simulink model "sigma2nd_d"  (Simulink 7.4)
settings: Solver=ode23t  StartTime=0.0  StopTime=70e-3  MaxStep=1e-6  RelTol=1e-3
PreLoadFcn:
  | Fs=512e3;
  | N=4;   % Number of CIC stages
  | R=16;  % Decimation factor
  | M=1;   % Delay order
  | b=ones(R*M,1)/(R*M);                % Compensate for gain of CIC for analysis purposes.
  | CICnum = conv(b,conv(b,conv(b,b)));  % overall cic numerator
  | load d4_coeff;
StartFcn:
  | tic
StopFcn:
  | trun=toc
undefined symbols (not defined in the file or in its folder): One, sided
libraries: powerlib x72, dspmlti4 x2, simulink x2, dspsnks4 x1
settings Model: Creator=dbenson  LastModifiedBy=Dick
settings DataIOCC: SaveOutput=off  SaveTime=off  SignalLoggingName=sigsOut
settings OptimizationCC: InlineInvariantSignals=on  InitFltsAndDblsToZero=on
settings DebuggingCC: SaveWithParameterizedLinksMsg=none  SignalResolutionControl=TryResolveAllWithWarning  SolverPrmCheckMsg=none  MultiTaskDSMMsg=warning  MultiTaskCondExecSysMsg=none  UnconnectedLineMsg=none  StrictBusMsg=None
settings HardwareCC: TargetUnknown=on
settings RTWCC: IncludeERTFirstTime=on
settings GRTTargetCC: TargetFcnLib=ansi_tfl_tmw.mat

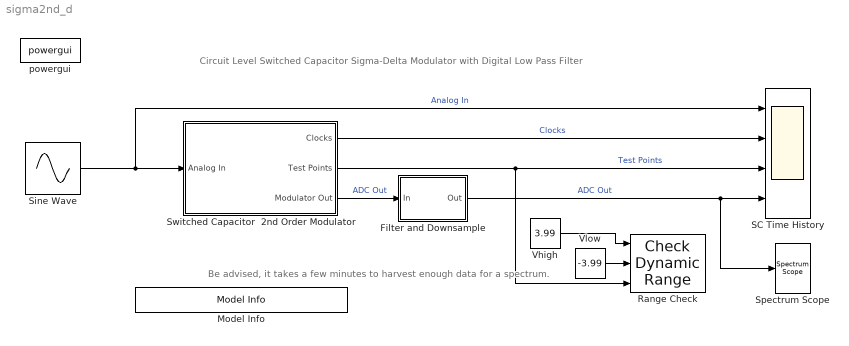
== system sigma2nd_d ==
  note: Circuit Level Switched Capacitor Sigma-Delta Modulator
      | with
      | Digital Low Pass Filter
  note: Be advised, it takes a few minutes
      |  to harvest enough data for a spectrum.
  Filter and Downsample : Subsystem
  Model Info : simulink/Model-Wide Utilities/Model Info  SystemSampleTime=-1  InitialBlockCM=None  BlockCM=None  Frame=on  DisplayStringWithTags=Copywrite 2005-2010 The MathWorks, Inc.  HorizontalTextAlignment=Center  LeftAlignmentValue=0.5  SourceBlockDiagram=sigma2nd_d  TagMaxNumber=20
  Range Check : simulink/Model Verification/Check  Dynamic Range  Description=min < sig < max  SystemSampleTime=-1  enabled=on  stopWhenAssertionFail=off  export=off  icon=graphic
  SC Time History : Scope  NumInputPorts=4
      settings: TimeRange=0.0025  YMin=-0.5~-0.2~-4~-0.5  YMax=0.5~1.2~4~0.5  DataFormat=Structure  Decimation=40
  Sine Wave : Sin  Amplitude=0.45  Bias=0  Frequency=500*2*pi  Phase=0  Samples=10  SampleTime=0  Offset=0
  Spectrum Scope : dspsnks4/Spectrum Scope  DialogController=dspdialog.SpectrumScope  DialogControllerArgs=DataTag2  SystemSampleTime=-1  ScopeProperties=on  Domain=Frequency  HorizSpan=1  UseBuffer=on  BufferSize=512  Overlap=0  inpFftLenInherit=off  FFTlength=128  numAvg=1  DisplayProperties=off  AxisGrid=on  Memory=off  FrameNumber=on  AxisLegend=off  AxisZoom=off  OpenScopeAtSimStart=on  OpenScopeImmediately=off  FigPos=[444 39 414 275]  AxisProperties=off  XUnits=Hertz  XRange=One-sided ([0...Fs/2])  XDisplay=0  InheritXIncr=on  XIncr=64/Fs  XLabel=Samples  XLimit=Auto  YUnits=dBW  XMax=1  XMin=0  YLabel=dBW  LineProperties=off  wintypeSpecScope=Hann  RsSpecScope=50  betaSpecScope=5  winsampSpecScope=Periodic  XAxisParamsVer=6.9
      settings: YMin=-100  YMax=0
  Switched Capacitor  2nd Order Modulator : Subsystem
  Vhigh : Constant  Value=3.99  OutDataType=sfix(16)  OutScaling=2^0
  Vlow : Constant  Value=-3.99  OutDataType=sfix(16)  OutScaling=2^0
  powergui : powerlib/powergui  SystemSampleTime=-1  SimulationMode=Continuous  SampleTime=50e-6  frequency=60  SPID=off  DisableSnubberDevices=off  DisableRonSwitches=off  DisableVfSwitches=off  SwTol=0  Interpol=off  frequencyindice=0  echomessages=off  HookPort=off  DisplayEquations=off  FunctionMessages=off  EnableUseOfTLC=off  x0status=blocks  RestoreLinks=warning  Frange=[0:2:500]  Ylog=off  Xlog=on  ShowGrid=off  save=off  variable=ZData  ZoomFFT=on  StartTime=0.0  cycles=1  DisplayStyle=1  fundamental=60  FreqAxis=off  MaxFrequency=1000  frequencyindicesteady=1  RmsSteady=1  display=off  Ts=0  methode=off
  wires:
  Sine Wave/1 -> Switched Capacitor  2nd Order Modulator/1(Analog In), SC Time History/1  "Analog In"
  Switched Capacitor  2nd Order Modulator/3(Modulator Out) -> Filter and Downsample/1(In)  "ADC Out"
  Switched Capacitor  2nd Order Modulator/2(Test Points) -> Range Check/3, SC Time History/3  "Test Points"
  Vhigh/1 -> Range Check/1
  Vlow/1 -> Range Check/2
  Switched Capacitor  2nd Order Modulator/1(Clocks) -> SC Time History/2  "Clocks"
  Filter and Downsample/1(Out) -> SC Time History/4, Spectrum Scope/1  "ADC Out"

== system sigma2nd_d/Filter and Downsample ==
  In : Inport  OutDataType=sfix(16)  OutScaling=2^0
  D=16 Cascaded Integrator Comb Filter : dspmlti4/FIR Decimation  DialogController=dspdialog.FIRDecimation  DialogControllerArgs=DataTag0  h=CICnum  D=16  filtStruct=Direct form  framing=Maintain input frame size  outputBufInitCond=0  roundingMode=Floor  overflowMode=off  FilterSource=Specify via dialog  FilterObject=Hm_firdecim
  "D=4 with inverse sinc correction " : dspmlti4/FIR Decimation  DialogController=dspdialog.FIRDecimation  DialogControllerArgs=DataTag1  h=d4_coeff  D=4  filtStruct=Direct form  framing=Maintain input frame size  outputBufInitCond=0  roundingMode=Floor  overflowMode=off  FilterSource=Specify via dialog  FilterObject=Hm_firdecim
  Out : Outport  OutDataType=sfix(16)  OutScaling=2^0
  wires:
  "D=4 with inverse sinc correction "/1 -> Out/1
  In/1 -> D=16 Cascaded Integrator Comb Filter/1
  D=16 Cascaded Integrator Comb Filter/1 -> "D=4 with inverse sinc correction "/1

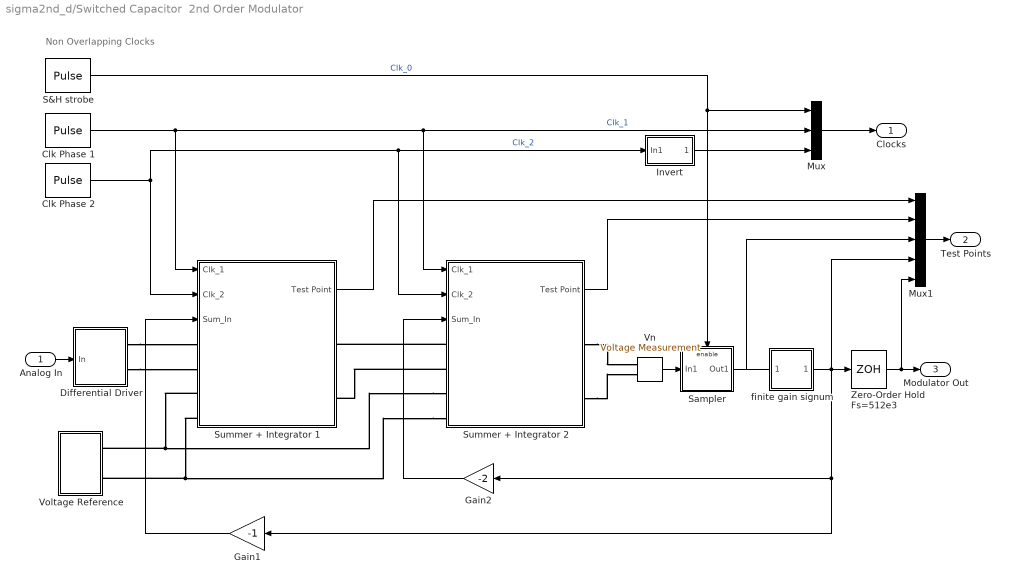
== system sigma2nd_d/Switched Capacitor  2nd Order Modulator ==
  note: Non Overlapping Clocks
  Analog In : Inport  OutDataType=sfix(16)  OutScaling=2^0
  Clk Phase 1 : DiscretePulseGenerator  PulseType=Time based  Amplitude=1  Period=1/Fs  PulseWidth=49.9  PhaseDelay=0.001/Fs  SampleTime=1
  Clk Phase 2 : DiscretePulseGenerator  PulseType=Time based  Amplitude=1  Period=1/Fs  PulseWidth=50.1  PhaseDelay=0  SampleTime=1
  Differential Driver : Subsystem
  Gain1 : Gain  Gain=-1  ParameterDataType=sfix(16)  ParameterScaling=2^0  OutDataType=sfix(16)  OutScaling=2^0  SaturateOnIntegerOverflow=on  OutDataTypeStr=Inherit: Same as input  ParamDataTypeStr=Inherit: Same as input
  Gain2 : Gain  Gain=-2  ParameterDataType=sfix(16)  ParameterScaling=2^0  OutDataType=sfix(16)  OutScaling=2^0  SaturateOnIntegerOverflow=on  OutDataTypeStr=Inherit: Same as input  ParamDataTypeStr=Inherit: Same as input
  Invert : Subsystem
  Mux : Mux  Inputs=3
  Mux1 : Mux  Inputs=5
  S&H strobe : DiscretePulseGenerator  PulseType=Time based  Amplitude=1  Period=1/Fs  PulseWidth=0.01  PhaseDelay=0.5005/Fs  SampleTime=1
  Sampler : Subsystem
  Summer + Integrator 1 : Subsystem
  Summer + Integrator 2 : Subsystem
  "Vn " : powerlib/Measurements/Voltage Measurement  Tag=PoWeRsYsTeMmEaSuReMeNt  DialogController=POWERSYS.PowerSysDialog  SystemSampleTime=-1  PhasorSimulation=off  OutputType=Magnitude  PSBequivalent=0
  Voltage Reference : Subsystem
  "Zero-Order Hold  Fs=512e3 " : ZeroOrderHold  SampleTime=1/Fs
  "finite gain signum " : Subsystem  mask{alpha=1e6}
      mask init:
      | x=-3:0.05:3;  y= tanh(alpha*x);
      mask Display: plot(x,y)
  Clocks : Outport  OutDataType=sfix(16)  OutScaling=2^0
  Test Points : Outport  Port=2  OutDataType=sfix(16)  OutScaling=2^0
  Modulator Out : Outport  Port=3  OutDataType=sfix(16)  OutScaling=2^0
  wires:
  Clk Phase 1/1 -> Summer + Integrator 1/1(Clk_1), Mux/2, Summer + Integrator 2/1(Clk_1)  "Clk_1"
  Clk Phase 2/1 -> Summer + Integrator 1/2(Clk_2), Summer + Integrator 2/2(Clk_2), Invert/1(In1)  "Clk_2"
  "Vn "/1 -> Sampler/1(In1)
  Gain1/1 -> Summer + Integrator 1/3(Sum_In)
  Analog In/1 -> Differential Driver/1(In)
  Mux/1 -> Clocks/1
  S&H strobe/1 -> Mux/1, Sampler/Enable  "Clk_0"
  Gain2/1 -> Summer + Integrator 2/3(Sum_In)
  Mux1/1 -> Test Points/1
  Sampler/1(Out1) -> "finite gain signum "/1(In1), Mux1/3
  "Zero-Order Hold  Fs=512e3 "/1 -> Modulator Out/1, Mux1/5
  Invert/1(Out1) -> Mux/3
  Summer + Integrator 1/1(Test Point) -> Mux1/1
  Summer + Integrator 2/1(Test Point) -> Mux1/2
  "finite gain signum "/1(Out1) -> Mux1/4, "Zero-Order Hold  Fs=512e3 "/1, Gain2/1, Gain1/1
  connections:
  Summer + Integrator 2/LConn3 -- Voltage Reference/RConn1 -- Summer + Integrator 1/LConn3
  Summer + Integrator 2/LConn4 -- Summer + Integrator 1/LConn4 -- Voltage Reference/RConn2
  Differential Driver/RConn1 -- Summer + Integrator 1/LConn1
  Differential Driver/RConn2 -- Summer + Integrator 1/LConn2
  Summer + Integrator 2/RConn2 -- "Vn "/LConn2
  Summer + Integrator 2/RConn1 -- "Vn "/LConn1
  Summer + Integrator 2/LConn1 -- Summer + Integrator 1/RConn1
  Summer + Integrator 2/LConn2 -- Summer + Integrator 1/RConn2

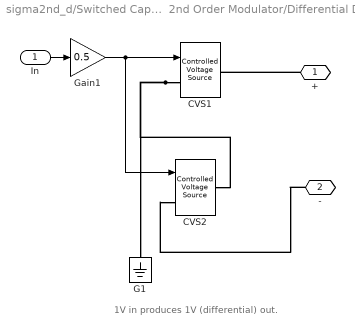
== system sigma2nd_d/Switched Capacitor  2nd Order Modulator/Differential Driver ==
  note: 1V in produces 1V (differential) out.
  In : Inport  OutDataType=sfix(16)  OutScaling=2^0
  CVS1 : powerlib/Electrical Sources/Controlled Voltage Source  Description=source block  DialogController=POWERSYS.PowerSysDialog  SystemSampleTime=-1  Initialize=off  Source_Type=AC  Amplitude=0  Phase=0  Frequency=0  Measurements=None
      settings: AttributesFormatString=\n
  CVS2 : powerlib/Electrical Sources/Controlled Voltage Source  Description=source block  DialogController=POWERSYS.PowerSysDialog  SystemSampleTime=-1  Initialize=off  Source_Type=AC  Amplitude=0  Phase=0  Frequency=0  Measurements=None
      settings: AttributesFormatString=\n
  G1 : powerlib/Elements/Ground  DialogController=POWERSYS.PowerSysDialog  PhysicalDomain=powersysdomain  SubClassName=unknown  LeftPortType=p1  RightPortType=p1  LConnTagsString=a
  Gain1 : Gain  Gain=0.5  ParameterDataType=sfix(16)  ParameterScaling=2^0  OutDataType=sfix(16)  OutScaling=2^0  SaturateOnIntegerOverflow=on  OutDataTypeStr=Inherit: Same as input  ParamDataTypeStr=Inherit: Same as input
  + : PMIOPort  Port=1  Side=Right
  - : PMIOPort  Port=2  Side=Right
  wires:
  In/1 -> Gain1/1
  Gain1/1 -> CVS1/1, CVS2/1
  connections:
  CVS1/LConn1 -- CVS2/RConn1 -- G1/LConn1
  +/RConn1 -- CVS1/RConn1
  -/RConn1 -- CVS2/LConn1

== system sigma2nd_d/Switched Capacitor  2nd Order Modulator/Invert ==
  In1 : Inport  OutDataType=sfix(16)  OutScaling=2^0
  Data Type Conversion : DataTypeConversion  OutDataTypeMode=boolean  OutDataType=sfix(16)  OutScaling=2^0  OutDataTypeStr=boolean  SaturateOnIntegerOverflow=on  RndMeth=Zero
  Data Type Conversion1 : DataTypeConversion  OutDataTypeMode=double  OutDataType=sfix(16)  OutScaling=2^0  OutDataTypeStr=double  SaturateOnIntegerOverflow=on  RndMeth=Zero
  Logical Operator : Logic  Operator=NOT  AllPortsSameDT=off
  Out1 : Outport  OutDataType=sfix(16)  OutScaling=2^0
  wires:
  Data Type Conversion/1 -> Logical Operator/1
  Logical Operator/1 -> Data Type Conversion1/1
  In1/1 -> Data Type Conversion/1
  Data Type Conversion1/1 -> Out1/1

== system sigma2nd_d/Switched Capacitor  2nd Order Modulator/Sampler ==
  In1 : Inport  OutDataType=sfix(16)  OutScaling=2^0
  Enable : EnablePort
  Out1 : Outport  OutDataType=sfix(16)  OutScaling=2^0  InitialOutput=[0]
  wires:
  In1/1 -> Out1/1

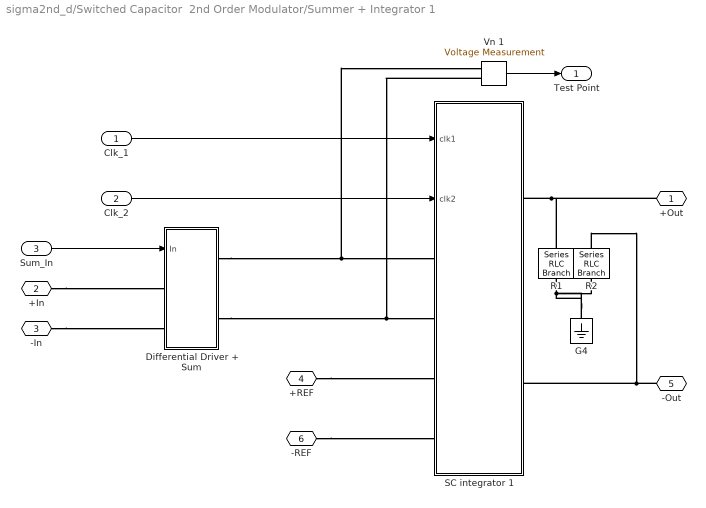
== system sigma2nd_d/Switched Capacitor  2nd Order Modulator/Summer + Integrator 1 ==
  Clk_1 : Inport  OutDataType=sfix(16)  OutScaling=2^0
  Clk_2 : Inport  Port=2  OutDataType=sfix(16)  OutScaling=2^0
  Sum_In : Inport  Port=3  OutDataType=sfix(16)  OutScaling=2^0
  Differential Driver + Sum : Subsystem
  G4 : powerlib/Elements/Ground  DialogController=POWERSYS.PowerSysDialog  PhysicalDomain=powersysdomain  SubClassName=unknown  LeftPortType=p1  RightPortType=p1  LConnTagsString=a
  R1 : powerlib/Elements/Series RLC Branch  DialogController=POWERSYS.PowerSysDialog  PhysicalDomain=powersysdomain  SubClassName=unknown  LeftPortType=p1  RightPortType=p1  LConnTagsString=__new0  RConnTagsString=__new0  BranchType=R  Resistance=1e9  Inductance=1.0  SetiL0=off  InitialCurrent=0  Capacitance=1.0  Setx0=off  InitialVoltage=0  Measurements=None
  R2 : powerlib/Elements/Series RLC Branch  DialogController=POWERSYS.PowerSysDialog  PhysicalDomain=powersysdomain  SubClassName=unknown  LeftPortType=p1  RightPortType=p1  LConnTagsString=__new0  RConnTagsString=__new0  BranchType=R  Resistance=1e9  Inductance=1.0  SetiL0=off  InitialCurrent=0  Capacitance=1.0  Setx0=off  InitialVoltage=0  Measurements=None
  SC integrator 1 : Subsystem  mask{Ci=4e-12, Cs=2e-12, Ron=10, Fb1=1e9, Fb2=1e8, Avol=2000, Vs=4, Slew=inf}
      mask prompts: Ci "integrating Cap"; Cs "Sampling Cap"; Ron "Switch on resistor"
  Vn 1 : powerlib/Measurements/Voltage Measurement  Tag=PoWeRsYsTeMmEaSuReMeNt  DialogController=POWERSYS.PowerSysDialog  SystemSampleTime=-1  PhasorSimulation=off  OutputType=Magnitude  PSBequivalent=0
  +Out : PMIOPort  Port=1  Side=Right
  +In : PMIOPort  Port=2  Side=Left
  -In : PMIOPort  Port=3  Side=Left
  +REF : PMIOPort  Port=4  Side=Left
  -Out : PMIOPort  Port=5  Side=Right
  -REF : PMIOPort  Port=6  Side=Left
  Test Point : Outport  OutDataType=sfix(16)  OutScaling=2^0
  wires:
  Clk_1/1 -> SC integrator 1/1(clk1)
  Clk_2/1 -> SC integrator 1/2(clk2)
  Sum_In/1 -> Differential Driver + Sum/1(In)
  Vn 1/1 -> Test Point/1
  connections:
  Differential Driver + Sum/RConn1 -- SC integrator 1/LConn1 -- Vn 1/LConn1
  Vn 1/LConn2 -- SC integrator 1/LConn2 -- Differential Driver + Sum/RConn2
  +Out/RConn1 -- SC integrator 1/RConn1 -- R1/RConn1
  +REF/RConn1 -- SC integrator 1/LConn3
  -Out/RConn1 -- SC integrator 1/RConn2 -- R2/RConn1
  -REF/RConn1 -- SC integrator 1/LConn4
  +In/RConn1 -- Differential Driver + Sum/LConn1
  -In/RConn1 -- Differential Driver + Sum/LConn2
  R1/LConn1 -- G4/LConn1 -- R2/LConn1

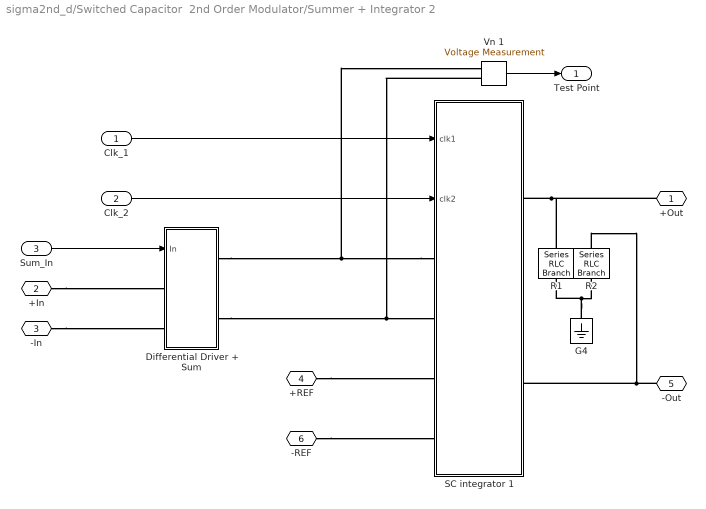
== system sigma2nd_d/Switched Capacitor  2nd Order Modulator/Summer + Integrator 2 ==
  Clk_1 : Inport  OutDataType=sfix(16)  OutScaling=2^0
  Clk_2 : Inport  Port=2  OutDataType=sfix(16)  OutScaling=2^0
  Sum_In : Inport  Port=3  OutDataType=sfix(16)  OutScaling=2^0
  Differential Driver + Sum : Subsystem
  G4 : powerlib/Elements/Ground  DialogController=POWERSYS.PowerSysDialog  PhysicalDomain=powersysdomain  SubClassName=unknown  LeftPortType=p1  RightPortType=p1  LConnTagsString=a
  R1 : powerlib/Elements/Series RLC Branch  DialogController=POWERSYS.PowerSysDialog  PhysicalDomain=powersysdomain  SubClassName=unknown  LeftPortType=p1  RightPortType=p1  LConnTagsString=__new0  RConnTagsString=__new0  BranchType=R  Resistance=1e9  Inductance=1.0  SetiL0=off  InitialCurrent=0  Capacitance=1.0  Setx0=off  InitialVoltage=0  Measurements=None
  R2 : powerlib/Elements/Series RLC Branch  DialogController=POWERSYS.PowerSysDialog  PhysicalDomain=powersysdomain  SubClassName=unknown  LeftPortType=p1  RightPortType=p1  LConnTagsString=__new0  RConnTagsString=__new0  BranchType=R  Resistance=1e9  Inductance=1.0  SetiL0=off  InitialCurrent=0  Capacitance=1.0  Setx0=off  InitialVoltage=0  Measurements=None
  SC integrator 1 : Subsystem  mask{Ci=4e-12, Cs=2e-12, Ron=10, Fb1=1e9, Fb2=1e8, Avol=2000, Vs=4, Slew=inf}
      mask prompts: Ci "integrating Cap"; Cs "Sampling Cap"; Ron "Switch on resistor"
  Vn 1 : powerlib/Measurements/Voltage Measurement  Tag=PoWeRsYsTeMmEaSuReMeNt  DialogController=POWERSYS.PowerSysDialog  SystemSampleTime=-1  PhasorSimulation=off  OutputType=Magnitude  PSBequivalent=0
  +Out : PMIOPort  Port=1  Side=Right
  +In : PMIOPort  Port=2  Side=Left
  -In : PMIOPort  Port=3  Side=Left
  +REF : PMIOPort  Port=4  Side=Left
  -Out : PMIOPort  Port=5  Side=Right
  -REF : PMIOPort  Port=6  Side=Left
  Test Point : Outport  OutDataType=sfix(16)  OutScaling=2^0
  wires:
  Vn 1/1 -> Test Point/1
  Sum_In/1 -> Differential Driver + Sum/1(In)
  Clk_2/1 -> SC integrator 1/2(clk2)
  Clk_1/1 -> SC integrator 1/1(clk1)
  connections:
  G4/LConn1 -- R1/LConn1 -- R2/LConn1
  -In/RConn1 -- Differential Driver + Sum/LConn2
  +In/RConn1 -- Differential Driver + Sum/LConn1
  -REF/RConn1 -- SC integrator 1/LConn4
  R2/RConn1 -- SC integrator 1/RConn2 -- -Out/RConn1
  +REF/RConn1 -- SC integrator 1/LConn3
  R1/RConn1 -- SC integrator 1/RConn1 -- +Out/RConn1
  Differential Driver + Sum/RConn2 -- SC integrator 1/LConn2 -- Vn 1/LConn2
  SC integrator 1/LConn1 -- Differential Driver + Sum/RConn1 -- Vn 1/LConn1

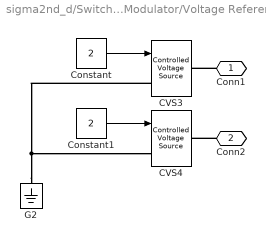
== system sigma2nd_d/Switched Capacitor  2nd Order Modulator/Voltage Reference ==
  CVS3 : powerlib/Electrical Sources/Controlled Voltage Source  Description=source block  DialogController=POWERSYS.PowerSysDialog  SystemSampleTime=-1  Initialize=off  Source_Type=AC  Amplitude=0  Phase=0  Frequency=0  Measurements=None
      settings: AttributesFormatString=\n
  CVS4 : powerlib/Electrical Sources/Controlled Voltage Source  Description=source block  DialogController=POWERSYS.PowerSysDialog  SystemSampleTime=-1  Initialize=off  Source_Type=AC  Amplitude=0  Phase=0  Frequency=0  Measurements=None
      settings: AttributesFormatString=\n
  Constant : Constant  Value=2  OutDataType=sfix(16)  OutScaling=2^0
  Constant1 : Constant  Value=2  OutDataType=sfix(16)  OutScaling=2^0
  G2 : powerlib/Elements/Ground  DialogController=POWERSYS.PowerSysDialog  PhysicalDomain=powersysdomain  SubClassName=unknown  LeftPortType=p1  RightPortType=p1  LConnTagsString=a
  Conn1 : PMIOPort  Port=1  Side=Right
  Conn2 : PMIOPort  Port=2  Side=Right
  wires:
  Constant/1 -> CVS3/1
  Constant1/1 -> CVS4/1
  connections:
  CVS3/LConn1 -- G2/LConn1 -- CVS4/LConn1
  Conn1/RConn1 -- CVS3/RConn1
  Conn2/RConn1 -- CVS4/RConn1

== system sigma2nd_d/Switched Capacitor  2nd Order Modulator/finite gain signum  ==
  In1 : Inport  OutDataType=sfix(16)  OutScaling=2^0
  Gain1 : Gain  Gain=alpha  ParameterDataType=sfix(16)  ParameterScaling=2^0  OutDataType=sfix(16)  OutScaling=2^0  SaturateOnIntegerOverflow=on  OutDataTypeStr=Inherit: Same as input  ParamDataTypeStr=Inherit: Same as input
  Hyperbolic Tangent : Trigonometry  Operator=tanh
  Memory : Memory
  Out1 : Outport  OutDataType=sfix(16)  OutScaling=2^0
  wires:
  In1/1 -> Gain1/1
  Gain1/1 -> Hyperbolic Tangent/1
  Hyperbolic Tangent/1 -> Memory/1
  Memory/1 -> Out1/1

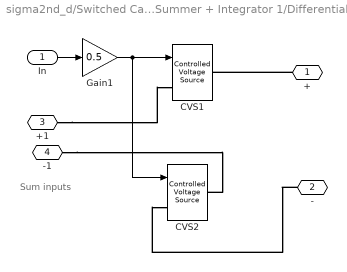
== system sigma2nd_d/Switched Capacitor  2nd Order Modulator/Summer + Integrator 1/Differential Driver + Sum ==
  note: Sum inputs
  In : Inport  OutDataType=sfix(16)  OutScaling=2^0
  CVS1 : powerlib/Electrical Sources/Controlled Voltage Source  Description=source block  DialogController=POWERSYS.PowerSysDialog  SystemSampleTime=-1  Initialize=off  Source_Type=AC  Amplitude=0  Phase=0  Frequency=0  Measurements=None
      settings: AttributesFormatString=\n
  CVS2 : powerlib/Electrical Sources/Controlled Voltage Source  Description=source block  DialogController=POWERSYS.PowerSysDialog  SystemSampleTime=-1  Initialize=off  Source_Type=AC  Amplitude=0  Phase=0  Frequency=0  Measurements=None
      settings: AttributesFormatString=\n
  Gain1 : Gain  Gain=0.5  ParameterDataType=sfix(16)  ParameterScaling=2^0  OutDataType=sfix(16)  OutScaling=2^0  SaturateOnIntegerOverflow=on  OutDataTypeStr=Inherit: Same as input  ParamDataTypeStr=Inherit: Same as input
  + : PMIOPort  Port=1  Side=Right
  - : PMIOPort  Port=2  Side=Right
  +1 : PMIOPort  Port=3  Side=Left
  -1 : PMIOPort  Port=4  Side=Left
  wires:
  In/1 -> Gain1/1
  Gain1/1 -> CVS1/1, CVS2/1
  connections:
  +/RConn1 -- CVS1/RConn1
  -/RConn1 -- CVS2/LConn1
  +1/RConn1 -- CVS1/LConn1
  -1/RConn1 -- CVS2/RConn1

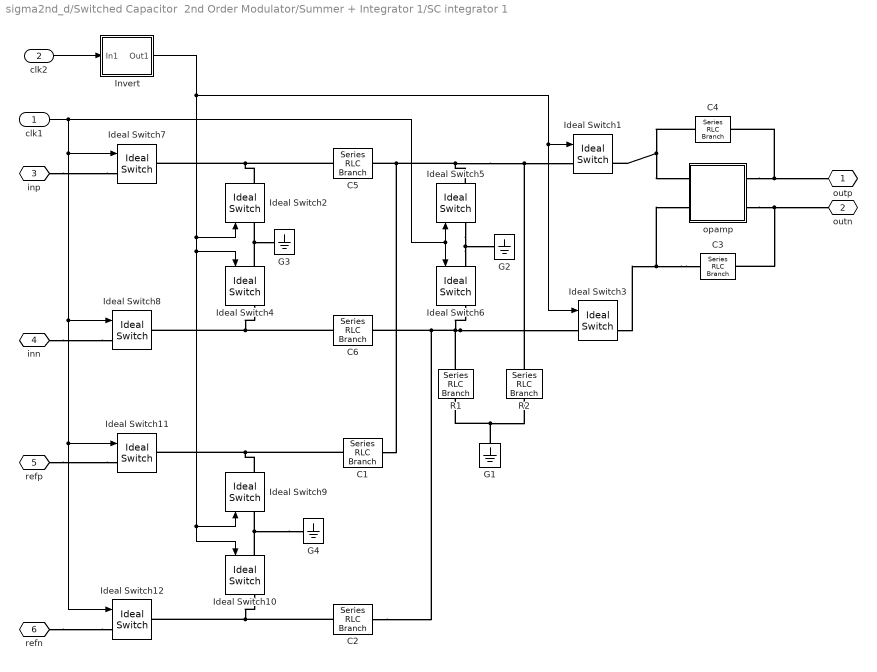
== system sigma2nd_d/Switched Capacitor  2nd Order Modulator/Summer + Integrator 1/SC integrator 1 ==
  clk1 : Inport  OutDataType=sfix(16)  OutScaling=2^0
  clk2 : Inport  Port=2  OutDataType=sfix(16)  OutScaling=2^0
  C{1..2,5..6} (4 alike) : powerlib/Elements/Series RLC Branch  DialogController=POWERSYS.PowerSysDialog  PhysicalDomain=powersysdomain  SubClassName=unknown  LeftPortType=p1  RightPortType=p1  LConnTagsString=__new0  RConnTagsString=__new0  BranchType=C  Resistance=1.0  Inductance=1.0  SetiL0=off  InitialCurrent=0  Capacitance=Cs  Setx0=off  InitialVoltage=0  Measurements=None
  C3 : powerlib/Elements/Series RLC Branch  DialogController=POWERSYS.PowerSysDialog  PhysicalDomain=powersysdomain  SubClassName=unknown  LeftPortType=p1  RightPortType=p1  LConnTagsString=__new0  RConnTagsString=__new0  BranchType=C  Resistance=1.0  Inductance=1.0  SetiL0=off  InitialCurrent=0  Capacitance=Ci  Setx0=off  InitialVoltage=0  Measurements=None
  "C4 " : powerlib/Elements/Series RLC Branch  DialogController=POWERSYS.PowerSysDialog  PhysicalDomain=powersysdomain  SubClassName=unknown  LeftPortType=p1  RightPortType=p1  LConnTagsString=__new0  RConnTagsString=__new0  BranchType=C  Resistance=1.0  Inductance=1.0  SetiL0=off  InitialCurrent=0  Capacitance=Ci  Setx0=off  InitialVoltage=0  Measurements=None
  G{1..4} (4 alike) : powerlib/Elements/Ground  DialogController=POWERSYS.PowerSysDialog  PhysicalDomain=powersysdomain  SubClassName=unknown  LeftPortType=p1  RightPortType=p1  LConnTagsString=a
  Ideal Switch{1..12} (12 alike) : powerlib/Power Electronics/Ideal Switch  DialogController=POWERSYS.PowerSysDialog  SystemSampleTime=-1  Ron=Ron  Lon=1e-9  IC=1  Rs=0  Cs=0  Measurements=off
      settings: AttributesFormatString=\n
  Invert : Subsystem
  R1 : powerlib/Elements/Series RLC Branch  DialogController=POWERSYS.PowerSysDialog  PhysicalDomain=powersysdomain  SubClassName=unknown  LeftPortType=p1  RightPortType=p1  LConnTagsString=__new0  RConnTagsString=__new0  BranchType=R  Resistance=1e9  Inductance=1.0  SetiL0=off  InitialCurrent=0  Capacitance=1.0  Setx0=off  InitialVoltage=0  Measurements=None
  R2 : powerlib/Elements/Series RLC Branch  DialogController=POWERSYS.PowerSysDialog  PhysicalDomain=powersysdomain  SubClassName=unknown  LeftPortType=p1  RightPortType=p1  LConnTagsString=__new0  RConnTagsString=__new0  BranchType=R  Resistance=1e9  Inductance=1.0  SetiL0=off  InitialCurrent=0  Capacitance=1.0  Setx0=off  InitialVoltage=0  Measurements=None
  opamp : Subsystem  mask{f2=Fb1, f1=Fb2, Av=Avol, v_min=-Vs, v_max=Vs, slew_rate=Slew}
      mask prompts: f2 "break freq 2 in Hz"; f1 "break freq 1 in Hz"; Av "Av (voltage gain)"; v_min "Min Output"; v_max "Max Output"; slew_rate "slew rate (v/s)"
      mask Display: plot([0 1 0 0] , [1 0 -1 1 ]); text(0.15,0.4,'+'); text(0.15,-0.4,'-');
  outp : PMIOPort  Port=1  Side=Right
  outn : PMIOPort  Port=2  Side=Right
  inp : PMIOPort  Port=3  Side=Left
  inn : PMIOPort  Port=4  Side=Left
  refp : PMIOPort  Port=5  Side=Left
  refn : PMIOPort  Port=6  Side=Left
  wires:
  Invert/1(Out1) -> Ideal Switch4/1, Ideal Switch9/1, Ideal Switch10/1, Ideal Switch2/1, Ideal Switch3/1, Ideal Switch1/1
  clk1/1 -> Ideal Switch12/1, Ideal Switch11/1, Ideal Switch8/1, Ideal Switch7/1, Ideal Switch5/1, Ideal Switch6/1
  clk2/1 -> Invert/1(In1)
  connections:
  refn/RConn1 -- Ideal Switch12/LConn1
  refp/RConn1 -- Ideal Switch11/LConn1
  inn/RConn1 -- Ideal Switch8/LConn1
  inp/RConn1 -- Ideal Switch7/LConn1
  G4/LConn1 -- Ideal Switch9/LConn1 -- Ideal Switch10/LConn1
  Ideal Switch2/LConn1 -- G3/LConn1 -- Ideal Switch4/LConn1
  Ideal Switch6/LConn1 -- G2/LConn1 -- Ideal Switch5/LConn1
  Ideal Switch11/RConn1 -- C1/LConn1 -- Ideal Switch9/RConn1
  Ideal Switch1/RConn1 -- opamp/LConn1 -- "C4 "/RConn1
  opamp/RConn1 -- outp/RConn1 -- "C4 "/LConn1
  C1/RConn1 -- C5/RConn1 -- Ideal Switch5/RConn1 -- Ideal Switch1/LConn1 -- R2/RConn1
  Ideal Switch2/RConn1 -- Ideal Switch7/RConn1 -- C5/LConn1
  C3/RConn1 -- opamp/LConn2 -- Ideal Switch3/RConn1
  opamp/RConn2 -- outn/RConn1 -- C3/LConn1
  Ideal Switch12/RConn1 -- C2/LConn1 -- Ideal Switch10/RConn1
  C2/RConn1 -- C6/RConn1 -- Ideal Switch6/RConn1 -- Ideal Switch3/LConn1 -- R1/RConn1
  Ideal Switch4/RConn1 -- Ideal Switch8/RConn1 -- C6/LConn1
  R2/LConn1 -- G1/LConn1 -- R1/LConn1

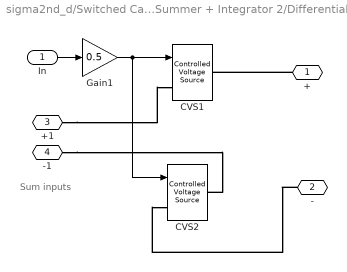
== system sigma2nd_d/Switched Capacitor  2nd Order Modulator/Summer + Integrator 2/Differential Driver + Sum ==
  note: Sum inputs
  In : Inport  OutDataType=sfix(16)  OutScaling=2^0
  CVS1 : powerlib/Electrical Sources/Controlled Voltage Source  Description=source block  DialogController=POWERSYS.PowerSysDialog  SystemSampleTime=-1  Initialize=off  Source_Type=AC  Amplitude=0  Phase=0  Frequency=0  Measurements=None
      settings: AttributesFormatString=\n
  CVS2 : powerlib/Electrical Sources/Controlled Voltage Source  Description=source block  DialogController=POWERSYS.PowerSysDialog  SystemSampleTime=-1  Initialize=off  Source_Type=AC  Amplitude=0  Phase=0  Frequency=0  Measurements=None
      settings: AttributesFormatString=\n
  Gain1 : Gain  Gain=0.5  ParameterDataType=sfix(16)  ParameterScaling=2^0  OutDataType=sfix(16)  OutScaling=2^0  SaturateOnIntegerOverflow=on  OutDataTypeStr=Inherit: Same as input  ParamDataTypeStr=Inherit: Same as input
  + : PMIOPort  Port=1  Side=Right
  - : PMIOPort  Port=2  Side=Right
  +1 : PMIOPort  Port=3  Side=Left
  -1 : PMIOPort  Port=4  Side=Left
  wires:
  Gain1/1 -> CVS2/1, CVS1/1
  In/1 -> Gain1/1
  connections:
  -1/RConn1 -- CVS2/RConn1
  +1/RConn1 -- CVS1/LConn1
  -/RConn1 -- CVS2/LConn1
  +/RConn1 -- CVS1/RConn1

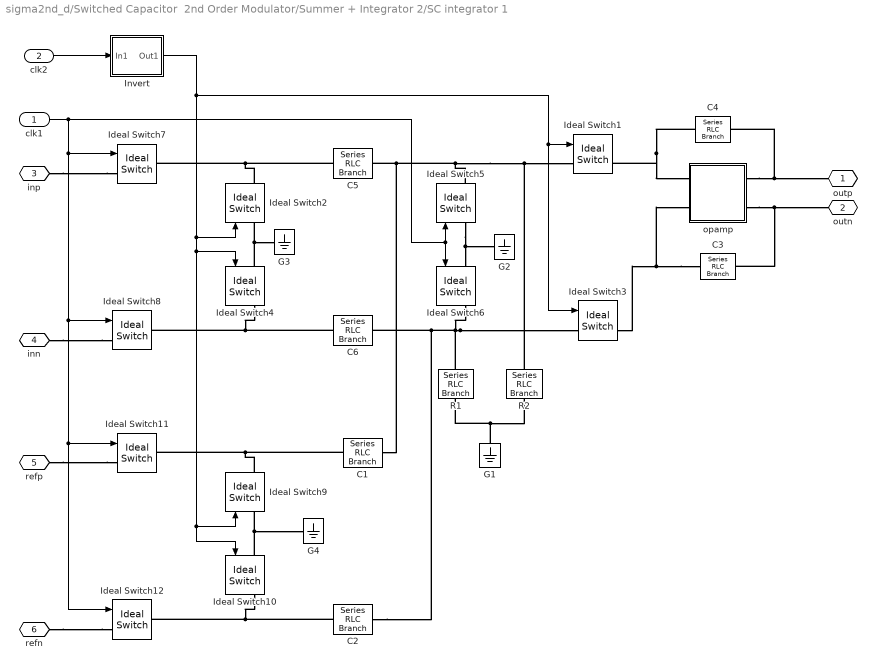
== system sigma2nd_d/Switched Capacitor  2nd Order Modulator/Summer + Integrator 2/SC integrator 1 ==
  clk1 : Inport  OutDataType=sfix(16)  OutScaling=2^0
  clk2 : Inport  Port=2  OutDataType=sfix(16)  OutScaling=2^0
  C{1..2,5..6} (4 alike) : powerlib/Elements/Series RLC Branch  DialogController=POWERSYS.PowerSysDialog  PhysicalDomain=powersysdomain  SubClassName=unknown  LeftPortType=p1  RightPortType=p1  LConnTagsString=__new0  RConnTagsString=__new0  BranchType=C  Resistance=1.0  Inductance=1.0  SetiL0=off  InitialCurrent=0  Capacitance=Cs  Setx0=off  InitialVoltage=0  Measurements=None
  C3 : powerlib/Elements/Series RLC Branch  DialogController=POWERSYS.PowerSysDialog  PhysicalDomain=powersysdomain  SubClassName=unknown  LeftPortType=p1  RightPortType=p1  LConnTagsString=__new0  RConnTagsString=__new0  BranchType=C  Resistance=1.0  Inductance=1.0  SetiL0=off  InitialCurrent=0  Capacitance=Ci  Setx0=off  InitialVoltage=0  Measurements=None
  "C4 " : powerlib/Elements/Series RLC Branch  DialogController=POWERSYS.PowerSysDialog  PhysicalDomain=powersysdomain  SubClassName=unknown  LeftPortType=p1  RightPortType=p1  LConnTagsString=__new0  RConnTagsString=__new0  BranchType=C  Resistance=1.0  Inductance=1.0  SetiL0=off  InitialCurrent=0  Capacitance=Ci  Setx0=off  InitialVoltage=0  Measurements=None
  G{1..4} (4 alike) : powerlib/Elements/Ground  DialogController=POWERSYS.PowerSysDialog  PhysicalDomain=powersysdomain  SubClassName=unknown  LeftPortType=p1  RightPortType=p1  LConnTagsString=a
  Ideal Switch{1..12} (12 alike) : powerlib/Power Electronics/Ideal Switch  DialogController=POWERSYS.PowerSysDialog  SystemSampleTime=-1  Ron=Ron  Lon=1e-9  IC=1  Rs=0  Cs=0  Measurements=off
      settings: AttributesFormatString=\n
  Invert : Subsystem
  R1 : powerlib/Elements/Series RLC Branch  DialogController=POWERSYS.PowerSysDialog  PhysicalDomain=powersysdomain  SubClassName=unknown  LeftPortType=p1  RightPortType=p1  LConnTagsString=__new0  RConnTagsString=__new0  BranchType=R  Resistance=1e9  Inductance=1.0  SetiL0=off  InitialCurrent=0  Capacitance=1.0  Setx0=off  InitialVoltage=0  Measurements=None
  R2 : powerlib/Elements/Series RLC Branch  DialogController=POWERSYS.PowerSysDialog  PhysicalDomain=powersysdomain  SubClassName=unknown  LeftPortType=p1  RightPortType=p1  LConnTagsString=__new0  RConnTagsString=__new0  BranchType=R  Resistance=1e9  Inductance=1.0  SetiL0=off  InitialCurrent=0  Capacitance=1.0  Setx0=off  InitialVoltage=0  Measurements=None
  opamp : Subsystem  mask{f2=Fb1, f1=Fb2, Av=Avol, v_min=-Vs, v_max=Vs, slew_rate=Slew}
      mask prompts: f2 "break freq 2 in Hz"; f1 "break freq 1 in Hz"; Av "Av (voltage gain)"; v_min "Min Output"; v_max "Max Output"; slew_rate "slew rate (v/s)"
      mask Display: plot([0 1 0 0] , [1 0 -1 1 ]); text(0.15,0.4,'+'); text(0.15,-0.4,'-');
  outp : PMIOPort  Port=1  Side=Right
  outn : PMIOPort  Port=2  Side=Right
  inp : PMIOPort  Port=3  Side=Left
  inn : PMIOPort  Port=4  Side=Left
  refp : PMIOPort  Port=5  Side=Left
  refn : PMIOPort  Port=6  Side=Left
  wires:
  clk2/1 -> Invert/1(In1)
  clk1/1 -> Ideal Switch6/1, Ideal Switch5/1, Ideal Switch7/1, Ideal Switch8/1, Ideal Switch11/1, Ideal Switch12/1
  Invert/1(Out1) -> Ideal Switch2/1, Ideal Switch10/1, Ideal Switch9/1, Ideal Switch4/1, Ideal Switch1/1, Ideal Switch3/1
  connections:
  R1/LConn1 -- G1/LConn1 -- R2/LConn1
  C6/LConn1 -- Ideal Switch8/RConn1 -- Ideal Switch4/RConn1
  R1/RConn1 -- Ideal Switch3/LConn1 -- Ideal Switch6/RConn1 -- C6/RConn1 -- C2/RConn1
  Ideal Switch10/RConn1 -- C2/LConn1 -- Ideal Switch12/RConn1
  C3/LConn1 -- outn/RConn1 -- opamp/RConn2
  Ideal Switch3/RConn1 -- opamp/LConn2 -- C3/RConn1
  C5/LConn1 -- Ideal Switch7/RConn1 -- Ideal Switch2/RConn1
  R2/RConn1 -- Ideal Switch1/LConn1 -- Ideal Switch5/RConn1 -- C5/RConn1 -- C1/RConn1
  "C4 "/LConn1 -- outp/RConn1 -- opamp/RConn1
  "C4 "/RConn1 -- opamp/LConn1 -- Ideal Switch1/RConn1
  Ideal Switch9/RConn1 -- C1/LConn1 -- Ideal Switch11/RConn1
  Ideal Switch5/LConn1 -- G2/LConn1 -- Ideal Switch6/LConn1
  Ideal Switch4/LConn1 -- G3/LConn1 -- Ideal Switch2/LConn1
  Ideal Switch10/LConn1 -- Ideal Switch9/LConn1 -- G4/LConn1
  inp/RConn1 -- Ideal Switch7/LConn1
  inn/RConn1 -- Ideal Switch8/LConn1
  refp/RConn1 -- Ideal Switch11/LConn1
  refn/RConn1 -- Ideal Switch12/LConn1

== system sigma2nd_d/Switched Capacitor  2nd Order Modulator/Summer + Integrator 1/SC integrator 1/Invert ==
  In1 : Inport  OutDataType=sfix(16)  OutScaling=2^0
  Data Type Conversion : DataTypeConversion  OutDataTypeMode=boolean  OutDataType=sfix(16)  OutScaling=2^0  OutDataTypeStr=boolean  SaturateOnIntegerOverflow=on  RndMeth=Zero
  Data Type Conversion1 : DataTypeConversion  OutDataTypeMode=double  OutDataType=sfix(16)  OutScaling=2^0  OutDataTypeStr=double  SaturateOnIntegerOverflow=on  RndMeth=Zero
  Logical Operator : Logic  Operator=NOT  AllPortsSameDT=off
  Out1 : Outport  OutDataType=sfix(16)  OutScaling=2^0
  wires:
  Data Type Conversion1/1 -> Out1/1
  In1/1 -> Data Type Conversion/1
  Logical Operator/1 -> Data Type Conversion1/1
  Data Type Conversion/1 -> Logical Operator/1

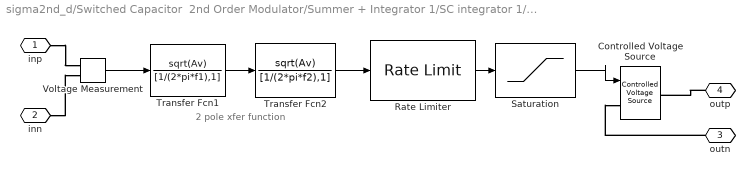
== system sigma2nd_d/Switched Capacitor  2nd Order Modulator/Summer + Integrator 1/SC integrator 1/opamp ==
  note: 2 pole xfer function
  Controlled Voltage Source : powerlib/Electrical Sources/Controlled Voltage Source  Description=source block  DialogController=POWERSYS.PowerSysDialog  SystemSampleTime=-1  Initialize=on  Source_Type=AC  Amplitude=0  Phase=0  Frequency=0  Measurements=None
      settings: AttributesFormatString=\n
  Rate Limiter : RateLimiter  RisingSlewLimit=slew_rate  FallingSlewLimit=-slew_rate
  Saturation : Saturate  UpperLimit=v_max  LowerLimit=v_min
  Transfer Fcn1 : TransferFcn  Numerator=sqrt(Av)  Denominator=[1/(2*pi*f1),1]
  Transfer Fcn2 : TransferFcn  Numerator=sqrt(Av)  Denominator=[1/(2*pi*f2),1]
  Voltage Measurement : powerlib/Measurements/Voltage Measurement  Tag=PoWeRsYsTeMmEaSuReMeNt  DialogController=POWERSYS.PowerSysDialog  SystemSampleTime=-1  PhasorSimulation=off  OutputType=Magnitude  PSBequivalent=0
  inp : PMIOPort  Port=1  Side=Left
  inn : PMIOPort  Port=2  Side=Left
  outn : PMIOPort  Port=3  Side=Right
  outp : PMIOPort  Port=4  Side=Right
  wires:
  Transfer Fcn2/1 -> Rate Limiter/1
  Voltage Measurement/1 -> Transfer Fcn1/1
  Saturation/1 -> Controlled Voltage Source/1
  Rate Limiter/1 -> Saturation/1
  Transfer Fcn1/1 -> Transfer Fcn2/1
  connections:
  outn/RConn1 -- Controlled Voltage Source/LConn1
  inn/RConn1 -- Voltage Measurement/LConn2
  outp/RConn1 -- Controlled Voltage Source/RConn1
  inp/RConn1 -- Voltage Measurement/LConn1

== system sigma2nd_d/Switched Capacitor  2nd Order Modulator/Summer + Integrator 2/SC integrator 1/Invert ==
  In1 : Inport  OutDataType=sfix(16)  OutScaling=2^0
  Data Type Conversion : DataTypeConversion  OutDataTypeMode=boolean  OutDataType=sfix(16)  OutScaling=2^0  OutDataTypeStr=boolean  SaturateOnIntegerOverflow=on  RndMeth=Zero
  Data Type Conversion1 : DataTypeConversion  OutDataTypeMode=double  OutDataType=sfix(16)  OutScaling=2^0  OutDataTypeStr=double  SaturateOnIntegerOverflow=on  RndMeth=Zero
  Logical Operator : Logic  Operator=NOT  AllPortsSameDT=off
  Out1 : Outport  OutDataType=sfix(16)  OutScaling=2^0
  wires:
  Data Type Conversion/1 -> Logical Operator/1
  Logical Operator/1 -> Data Type Conversion1/1
  In1/1 -> Data Type Conversion/1
  Data Type Conversion1/1 -> Out1/1

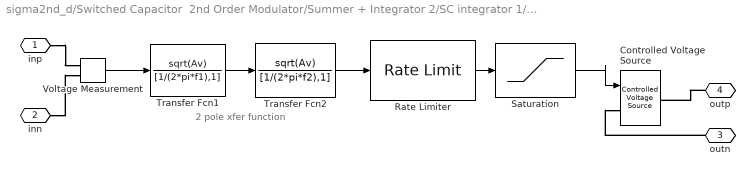
== system sigma2nd_d/Switched Capacitor  2nd Order Modulator/Summer + Integrator 2/SC integrator 1/opamp ==
  note: 2 pole xfer function
  Controlled Voltage Source : powerlib/Electrical Sources/Controlled Voltage Source  Description=source block  DialogController=POWERSYS.PowerSysDialog  SystemSampleTime=-1  Initialize=on  Source_Type=AC  Amplitude=0  Phase=0  Frequency=0  Measurements=None
      settings: AttributesFormatString=\n
  Rate Limiter : RateLimiter  RisingSlewLimit=slew_rate  FallingSlewLimit=-slew_rate
  Saturation : Saturate  UpperLimit=v_max  LowerLimit=v_min
  Transfer Fcn1 : TransferFcn  Numerator=sqrt(Av)  Denominator=[1/(2*pi*f1),1]
  Transfer Fcn2 : TransferFcn  Numerator=sqrt(Av)  Denominator=[1/(2*pi*f2),1]
  Voltage Measurement : powerlib/Measurements/Voltage Measurement  Tag=PoWeRsYsTeMmEaSuReMeNt  DialogController=POWERSYS.PowerSysDialog  SystemSampleTime=-1  PhasorSimulation=off  OutputType=Magnitude  PSBequivalent=0
  inp : PMIOPort  Port=1  Side=Left
  inn : PMIOPort  Port=2  Side=Left
  outn : PMIOPort  Port=3  Side=Right
  outp : PMIOPort  Port=4  Side=Right
  wires:
  Transfer Fcn1/1 -> Transfer Fcn2/1
  Rate Limiter/1 -> Saturation/1
  Saturation/1 -> Controlled Voltage Source/1
  Voltage Measurement/1 -> Transfer Fcn1/1
  Transfer Fcn2/1 -> Rate Limiter/1
  connections:
  inp/RConn1 -- Voltage Measurement/LConn1
  outp/RConn1 -- Controlled Voltage Source/RConn1
  inn/RConn1 -- Voltage Measurement/LConn2
  outn/RConn1 -- Controlled Voltage Source/LConn1
